simulink model "JointSpaceControl_own_MCP"  (R2013a)
settings: Solver=ode45  StartTime=0.0  StopTime=sim_end  MaxStep=0.008  RelTol=1e-3
PreLoadFcn:
  | Initialization
InitFcn:
  | Initialization
values from neighbouring files (symbols this model uses):
  a_max = [27 27 27 27 27 27]    [Initialization.m]
  dq_0 = qd_actual.signals.values(1,:)    [Initialization.m]
  K_0 = [            omega_1, zeros(1,5);         0,          omega_2, zeros(1,4);         zeros(1,2), omega_3, zeros(1,3);         zeros(1,3), omega_4, zeros(1,2);         zeros(1,4), omega_5, 0;         zeros(1,5), omega_6]    [Initialization.m]
  K_1 = [            omega_7, zeros(1,5);         0,          omega_8, zeros(1,4);         zeros(1,2), omega_9, zeros(1,3);         zeros(1,3), omega_10, zeros(1,2);         zeros(1,4), omega_11, 0;         zeros(1,5), omega_12]    [Initialization.m]
  q_0 = q_actual.signals.values(1,:)    [Initialization.m]
  q_max = 2*pi*ones(1,6)    [Initialization.m]
  q_min = -2*pi*ones(1,6)    [Initialization.m]
  torque_max = [150 150 150 28 28 28]    [Initialization.m]
  v_max = 3.4*ones(1,6)    [Initialization.m]
(part 1 of 4)
settings Model: Creator=kasiunia  LastModifiedBy=kasiunia

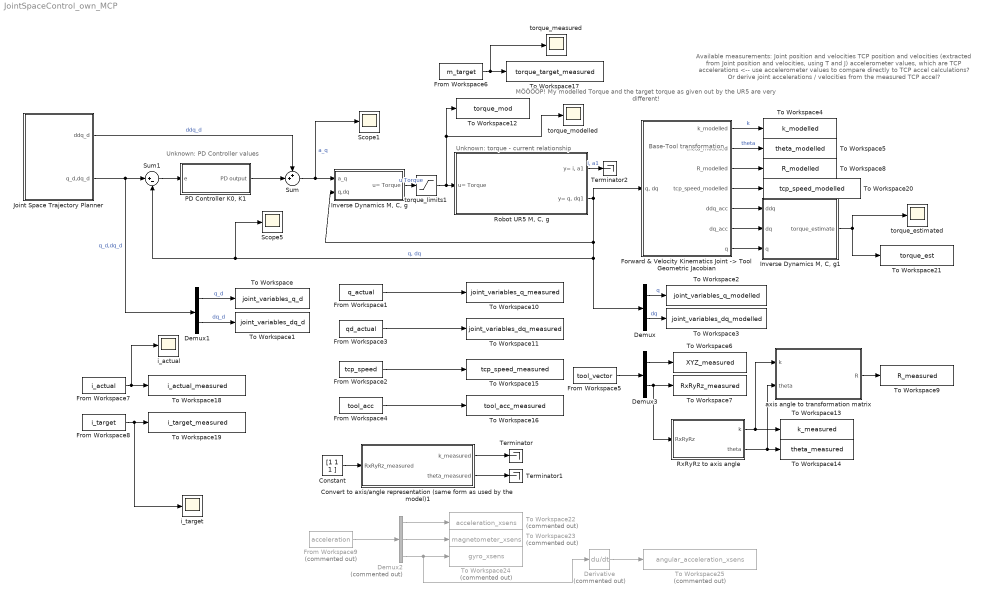
== system JointSpaceControl_own_MCP ==
  note: Base-Tool transformation
  note: Unknown: torque - current relationship
  note: Unknown: PD Controller values
  note: Available measurements:
      | Joint position and velocities
      | TCP position and velocities (extracted from Joint position and velocities,
      | using T and J)
      | accelerometer values, which are TCP accelerations
      | <-- use accelerometer values to compare directly to TCP accel calculations?
      | Or derive joint accelerations / velocities from the measured TCP accel?
  note: MÖÖÖÖP!
      | My modelled Torque and the target torque
      | as given out by the UR5 are very different!
  Constant : Constant  Value=[1 1 1 ]
  Convert to axis/angle representation (same form as used by the model)1 : Subsystem
  Demux : Demux  Outputs=[6 6]
  Demux1 : Demux  Outputs=[6 6]
  Demux2 : Demux  Commented=on  Outputs=[3 3 3]
  Demux3 : Demux  Outputs=[3 3]
  Derivative : Derivative  Commented=on
  "Forward & Velocity Kinematics Joint -> Tool Geometric Jacobian" : Subsystem
  From Workspace1 : FromWorkspace  VariableName=q_actual  SampleTime=0  OutputAfterFinalValue=Holding final value
  From Workspace2 : FromWorkspace  VariableName=tcp_speed  SampleTime=0  OutputAfterFinalValue=Setting to zero
  From Workspace3 : FromWorkspace  VariableName=qd_actual  SampleTime=0  OutputAfterFinalValue=Setting to zero
  From Workspace4 : FromWorkspace  VariableName=tool_acc  SampleTime=0  OutputAfterFinalValue=Setting to zero
  From Workspace5 : FromWorkspace  VariableName=tool_vector  SampleTime=0  OutputAfterFinalValue=Holding final value
  From Workspace6 : FromWorkspace  VariableName=m_target  SampleTime=0  OutputAfterFinalValue=Holding final value
  From Workspace7 : FromWorkspace  VariableName=i_actual  SampleTime=0  OutputAfterFinalValue=Holding final value
  From Workspace8 : FromWorkspace  VariableName=i_target  SampleTime=0  OutputAfterFinalValue=Holding final value
  From Workspace9 : FromWorkspace  Commented=on  VariableName=acceleration  SampleTime=0  OutputAfterFinalValue=Setting to zero
  "Inverse Dynamics M, C, g" : Subsystem
  "Inverse Dynamics M, C, g1" : Subsystem
  Joint Space Trajectory Planner : Subsystem
  "PD Controller K0, K1" : Subsystem
  "Robot UR5 M, C, g" : Subsystem
  RxRyRz to axis angle : MATLAB Function  TreatAsAtomicUnit=on
  Scope1 : Scope
      settings: ShowLegends=on
  Scope5 : Scope
      settings: ShowLegends=on  SaveName=ScopeData4
  Sum : Sum  Inputs=++|
  Sum1 : Sum  Inputs=|+-
  Terminator : Terminator
  Terminator1 : Terminator
  Terminator2 : Terminator
  To Workspace : ToWorkspace  VariableName=joint_variables_q_d  SampleTime=-1  SaveFormat=Timeseries
  To Workspace1 : ToWorkspace  VariableName=joint_variables_dq_d  SampleTime=-1  SaveFormat=Timeseries
  To Workspace10 : ToWorkspace  VariableName=joint_variables_q_measured  SampleTime=-1  SaveFormat=Timeseries
  To Workspace11 : ToWorkspace  VariableName=joint_variables_dq_measured  SampleTime=-1  SaveFormat=Timeseries
  To Workspace12 : ToWorkspace  VariableName=torque_mod  SampleTime=-1  SaveFormat=Timeseries
  To Workspace13 : ToWorkspace  VariableName=k_measured  SampleTime=-1  SaveFormat=Timeseries
  To Workspace14 : ToWorkspace  VariableName=theta_measured  SampleTime=-1  SaveFormat=Timeseries
  To Workspace15 : ToWorkspace  VariableName=tcp_speed_measured  SampleTime=-1  SaveFormat=Timeseries
  To Workspace16 : ToWorkspace  VariableName=tool_acc_measured  SampleTime=-1  SaveFormat=Timeseries
  To Workspace17 : ToWorkspace  VariableName=torque_target_measured  SampleTime=-1  SaveFormat=Timeseries
  To Workspace18 : ToWorkspace  VariableName=i_actual_measured  SampleTime=-1  SaveFormat=Timeseries
  To Workspace19 : ToWorkspace  VariableName=i_target_measured  SampleTime=-1  SaveFormat=Timeseries
  To Workspace2 : ToWorkspace  VariableName=joint_variables_q_modelled  SampleTime=-1  SaveFormat=Timeseries
  To Workspace20 : ToWorkspace  VariableName=tcp_speed_modelled  SampleTime=-1  SaveFormat=Timeseries
  To Workspace21 : ToWorkspace  VariableName=torque_est  SampleTime=-1  SaveFormat=Timeseries
  To Workspace22 : ToWorkspace  Commented=on  VariableName=acceleration_xsens  SampleTime=-1  SaveFormat=Timeseries
  To Workspace23 : ToWorkspace  Commented=on  VariableName=magnetometer_xsens  SampleTime=-1  SaveFormat=Timeseries
  To Workspace24 : ToWorkspace  Commented=on  VariableName=gyro_xsens  SampleTime=-1  SaveFormat=Timeseries
  To Workspace25 : ToWorkspace  Commented=on  VariableName=angular_acceleration_xsens  SampleTime=-1  SaveFormat=Timeseries
  To Workspace3 : ToWorkspace  VariableName=joint_variables_dq_modelled  SampleTime=-1  SaveFormat=Timeseries
  To Workspace4 : ToWorkspace  VariableName=k_modelled  SampleTime=-1  SaveFormat=Timeseries
  To Workspace5 : ToWorkspace  VariableName=theta_modelled  SampleTime=-1  SaveFormat=Timeseries
  To Workspace6 : ToWorkspace  VariableName=XYZ_measured  SampleTime=-1  SaveFormat=Timeseries
  To Workspace7 : ToWorkspace  VariableName=RxRyRz_measured  SampleTime=-1  SaveFormat=Timeseries
  To Workspace8 : ToWorkspace  VariableName=R_modelled  SampleTime=-1  SaveFormat=Timeseries
  To Workspace9 : ToWorkspace  VariableName=R_measured  SampleTime=-1  SaveFormat=Timeseries
  axis angle to transformation matrix : MATLAB Function  TreatAsAtomicUnit=on
  i_actual : Scope
      settings: ShowLegends=on  SaveName=ScopeData12
  i_target : Scope
      settings: SaveName=ScopeData13
  torque_estimated : Scope
      settings: ShowLegends=on  TimeRange=30  SaveName=ScopeData15
  torque_limits1 : Saturate  UpperLimit=torque_max  LowerLimit=-torque_max
  torque_measured : Scope
      settings: ShowLegends=on  TimeRange=50  SaveName=ScopeData16
  torque_modelled : Scope
      settings: ShowLegends=on  TimeRange=27.53110288501713  YMin=-0.9845613223672318  YMax=1.015679985521526  SaveName=ScopeData17
  wires:
  Sum/1 -> "Inverse Dynamics M, C, g"/1(a_q), Scope1/1  "a_q"
  "PD Controller K0, K1"/1(PD output) -> Sum/2
  Joint Space Trajectory Planner/2(q_d,dq_d) -> Sum1/1, Demux1/1  "q_d,dq_d"
  Sum1/1 -> "PD Controller K0, K1"/1(e)
  "Robot UR5 M, C, g"/2("y= q, dq1") -> Demux/1, Scope5/1, Sum1/2, "Inverse Dynamics M, C, g"/2(q,dq), "Forward & Velocity Kinematics Joint -> Tool Geometric Jacobian"/1("q, dq")  "q, dq"
  Joint Space Trajectory Planner/1(ddq_d) -> Sum/1  "ddq_d"
  Demux1/1 -> To Workspace/1  "q_d"
  Demux1/2 -> To Workspace1/1  "dq_d"
  Demux/1 -> To Workspace2/1  "q"
  Demux/2 -> To Workspace3/1  "dq"
  From Workspace5/1 -> Demux3/1
  Demux3/1 -> To Workspace6/1
  Demux3/2 -> RxRyRz to axis angle/1(RxRyRz), To Workspace7/1
  "Forward & Velocity Kinematics Joint -> Tool Geometric Jacobian"/1(k_modelled) -> To Workspace4/1  "k"
  "Forward & Velocity Kinematics Joint -> Tool Geometric Jacobian"/2(theta_modelled) -> To Workspace5/1  "theta"
  RxRyRz to axis angle/1(k) -> axis angle to transformation matrix/1(k), To Workspace13/1
  RxRyRz to axis angle/2(theta) -> axis angle to transformation matrix/2(theta), To Workspace14/1
  Constant/1 -> Convert to axis/angle representation (same form as used by the model)1/1(RxRyRz_measured)
  Convert to axis/angle representation (same form as used by the model)1/1(k_measured) -> Terminator/1
  Convert to axis/angle representation (same form as used by the model)1/2(theta_measured) -> Terminator1/1
  "Forward & Velocity Kinematics Joint -> Tool Geometric Jacobian"/3(R_modelled) -> To Workspace8/1
  axis angle to transformation matrix/1(R) -> To Workspace9/1
  "Robot UR5 M, C, g"/1("y= i, a1") -> Terminator2/1  "i, a1"
  From Workspace2/1 -> To Workspace15/1
  From Workspace4/1 -> To Workspace16/1
  From Workspace6/1 -> torque_measured/1, To Workspace17/1
  From Workspace7/1 -> i_actual/1, To Workspace18/1
  From Workspace8/1 -> i_target/1, To Workspace19/1
  "Forward & Velocity Kinematics Joint -> Tool Geometric Jacobian"/4(tcp_speed_modelled) -> To Workspace20/1
  "Forward & Velocity Kinematics Joint -> Tool Geometric Jacobian"/5(ddq_acc) -> "Inverse Dynamics M, C, g1"/1(ddq)
  "Forward & Velocity Kinematics Joint -> Tool Geometric Jacobian"/6(dq_acc) -> "Inverse Dynamics M, C, g1"/2(dq)
  "Inverse Dynamics M, C, g1"/1(torque_estimate) -> To Workspace21/1, torque_estimated/1
  "Forward & Velocity Kinematics Joint -> Tool Geometric Jacobian"/7(q) -> "Inverse Dynamics M, C, g1"/3(q)
  From Workspace9/1 -> Demux2/1
  Demux2/1 -> To Workspace22/1
  Demux2/2 -> To Workspace23/1
  Demux2/3 -> Derivative/1, To Workspace24/1
  Derivative/1 -> To Workspace25/1
  "Inverse Dynamics M, C, g"/1(u= Torque) -> torque_limits1/1  "u Torque"
  torque_limits1/1 -> torque_modelled/1, To Workspace12/1, "Robot UR5 M, C, g"/1(u= Torque)
  From Workspace1/1 -> To Workspace10/1
  From Workspace3/1 -> To Workspace11/1

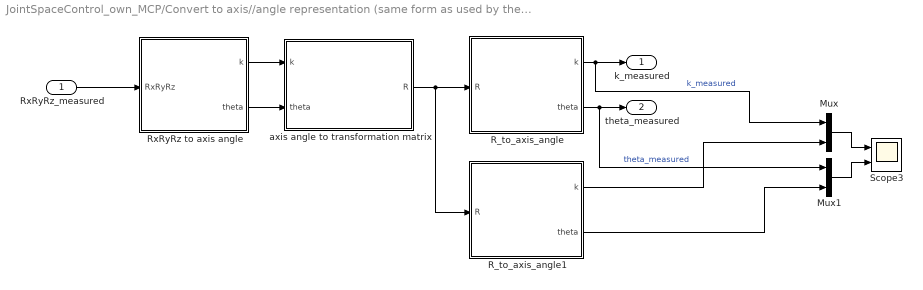
== system JointSpaceControl_own_MCP/Convert to axis//angle representation (same form as used by the model)1 ==
  RxRyRz_measured : Inport
  Mux : Mux  Inputs=[3 3]
  Mux1 : Mux  Inputs=2
  R_to_axis_angle : MATLAB Function  TreatAsAtomicUnit=on
  R_to_axis_angle1 : MATLAB Function  TreatAsAtomicUnit=on
  RxRyRz to axis angle : MATLAB Function  TreatAsAtomicUnit=on
  Scope3 : Scope  NumInputPorts=2
      settings: ShowLegends=on  YMin=-5~-5  YMax=5~5  SaveName=ScopeData6
  axis angle to transformation matrix : MATLAB Function  TreatAsAtomicUnit=on
  k_measured : Outport
  theta_measured : Outport  Port=2
  wires:
  R_to_axis_angle1/2(theta) -> Mux1/2
  R_to_axis_angle1/1(k) -> Mux/2
  Mux1/1 -> Scope3/2
  Mux/1 -> Scope3/1
  RxRyRz_measured/1 -> RxRyRz to axis angle/1(RxRyRz)
  RxRyRz to axis angle/2(theta) -> axis angle to transformation matrix/2(theta)
  RxRyRz to axis angle/1(k) -> axis angle to transformation matrix/1(k)
  R_to_axis_angle/1(k) -> k_measured/1, Mux/1  "k_measured"
  axis angle to transformation matrix/1(R) -> R_to_axis_angle/1(R), R_to_axis_angle1/1(R)
  R_to_axis_angle/2(theta) -> theta_measured/1, Mux1/1  "theta_measured"

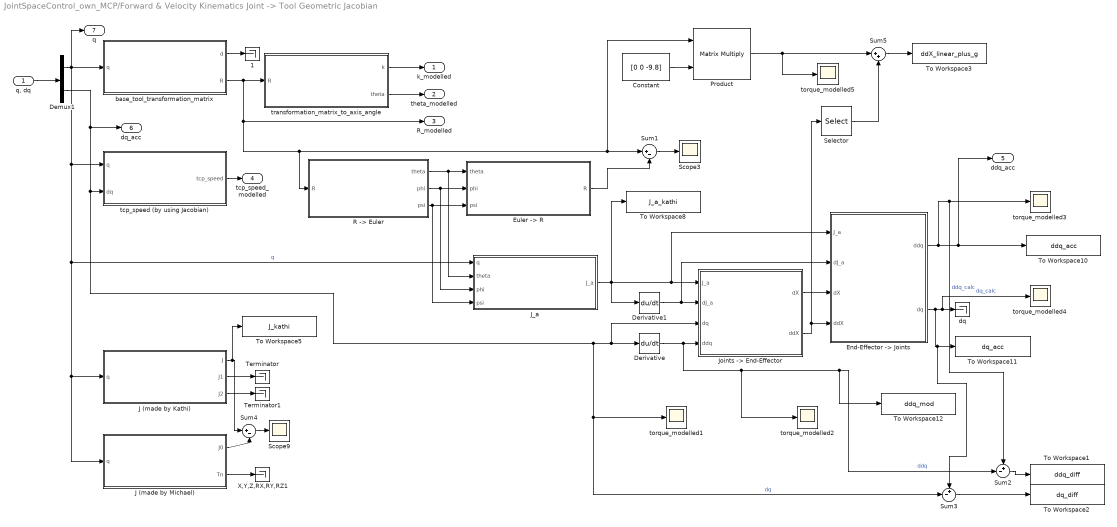
== system JointSpaceControl_own_MCP/Forward & Velocity Kinematics Joint -> Tool Geometric Jacobian ==
  "q, dq" : Inport
  1 : Terminator
  Constant : Constant  Value=[0 0 -9.8]
  Demux1 : Demux  Outputs=[6 6]
  Derivative : Derivative
  Derivative1 : Derivative
  "End-Effector -> Joints" : Subsystem
  "Euler -> R" : MATLAB Function  TreatAsAtomicUnit=on
  J (made by Kathi) : MATLAB Function  TreatAsAtomicUnit=on
  J (made by Michael) : MATLAB Function  TreatAsAtomicUnit=on
  J_a : MATLAB Function  TreatAsAtomicUnit=on
  "Joints -> End-Effector" : Subsystem
  Product : Product  Multiplication=Matrix(*)
  "R -> Euler" : MATLAB Function  TreatAsAtomicUnit=on
  Scope3 : Scope
      settings: ShowLegends=on  SaveName=ScopeData8
  Scope9 : Scope
      settings: ShowLegends=on  SaveName=ScopeData14
  Selector : Selector  InputPortWidth=6  IndexOptions=Index vector (dialog)  Indices=[1 2 3]  OutputSizes=1
  Sum1 : Sum  Inputs=|+-
  Sum2 : Sum  Inputs=+-|
  Sum3 : Sum  Inputs=+-|
  Sum4 : Sum  Inputs=|+-
  Sum5 : Sum  Inputs=|++
  Terminator : Terminator
  Terminator1 : Terminator
  To Workspace1 : ToWorkspace  VariableName=ddq_diff  SampleTime=-1  SaveFormat=Timeseries
  To Workspace10 : ToWorkspace  VariableName=ddq_acc  SampleTime=-1  SaveFormat=Timeseries
  To Workspace11 : ToWorkspace  VariableName=dq_acc  SampleTime=-1  SaveFormat=Timeseries
  To Workspace12 : ToWorkspace  VariableName=ddq_mod  SampleTime=-1  SaveFormat=Timeseries
  To Workspace2 : ToWorkspace  VariableName=dq_diff  SampleTime=-1  SaveFormat=Timeseries
  To Workspace3 : ToWorkspace  VariableName=ddX_linear_plus_g  SampleTime=-1  SaveFormat=Timeseries
  To Workspace5 : ToWorkspace  VariableName=J_kathi  SampleTime=-1  SaveFormat=Timeseries
  To Workspace8 : ToWorkspace  VariableName=J_a_kathi  SampleTime=-1  SaveFormat=Timeseries
  X,Y,Z,RX,RY,RZ1 : Terminator
  base_tool_transformation_matrix : MATLAB Function  TreatAsAtomicUnit=on
  dq : Terminator
  tcp_speed (by using Jacobian) : MATLAB Function  TreatAsAtomicUnit=on
  torque_modelled{1..5} (5 alike) : Scope
      torque_modelled1 settings: ShowLegends=on  SaveName=ScopeData5
      torque_modelled2 settings: ShowLegends=on  SaveName=ScopeData7
      torque_modelled3 settings: ShowLegends=on  SaveName=ScopeData9
      torque_modelled4 settings: ShowLegends=on  SaveName=ScopeData10
      torque_modelled5 settings: ShowLegends=on  SaveName=ScopeData11
  transformation_matrix_to_axis_angle : MATLAB Function  TreatAsAtomicUnit=on
  k_modelled : Outport
  theta_modelled : Outport  Port=2
  R_modelled : Outport  Port=3
  tcp_speed_modelled : Outport  Port=4
  ddq_acc : Outport  Port=5
  dq_acc : Outport  Port=6
  q : Outport  Port=7
  wires:
  "q, dq"/1 -> Demux1/1
  Demux1/1 -> q/1, J (made by Michael)/1(q), J (made by Kathi)/1(q), J_a/1(q), tcp_speed (by using Jacobian)/1(q), base_tool_transformation_matrix/1(q)  "q"
  Demux1/2 -> dq_acc/1, Sum3/2, torque_modelled1/1, "Joints -> End-Effector"/3(dq), Derivative/1, tcp_speed (by using Jacobian)/2(dq)  "dq"
  base_tool_transformation_matrix/2(R) -> transformation_matrix_to_axis_angle/1(R), Product/1, Sum1/1, "R -> Euler"/1(R), R_modelled/1
  transformation_matrix_to_axis_angle/1(k) -> k_modelled/1
  transformation_matrix_to_axis_angle/2(theta) -> theta_modelled/1
  J (made by Kathi)/1(J) -> To Workspace5/1, Sum4/1
  J (made by Michael)/1(J0) -> Sum4/2
  Sum4/1 -> Scope9/1
  J (made by Michael)/2(Tn) -> X,Y,Z,RX,RY,RZ1/1
  tcp_speed (by using Jacobian)/1(tcp_speed) -> tcp_speed_modelled/1
  "R -> Euler"/3(psi) -> J_a/4(psi), "Euler -> R"/3(psi)
  "R -> Euler"/2(phi) -> J_a/3(phi), "Euler -> R"/2(phi)
  "R -> Euler"/1(theta) -> J_a/2(theta), "Euler -> R"/1(theta)
  Sum1/1 -> Scope3/1
  base_tool_transformation_matrix/1(d) -> 1/1
  "Euler -> R"/1(R) -> Sum1/2
  J_a/1(J_a) -> "Joints -> End-Effector"/1(J_a), "End-Effector -> Joints"/1(J_a), To Workspace8/1, Derivative1/1
  Derivative/1 -> torque_modelled2/1, To Workspace12/1, Sum2/2, "Joints -> End-Effector"/4(ddq)  "ddq"
  "Joints -> End-Effector"/2(ddX) -> Selector/1, "End-Effector -> Joints"/4(ddX)
  "Joints -> End-Effector"/1(dX) -> "End-Effector -> Joints"/3(dX)
  Derivative1/1 -> "Joints -> End-Effector"/2(dJ_a), "End-Effector -> Joints"/2(dJ_a)
  "End-Effector -> Joints"/2(dq) -> Sum3/1, To Workspace11/1, torque_modelled4/1, dq/1  "dq_calc"
  J (made by Kathi)/2(J1) -> Terminator/1
  J (made by Kathi)/3(J2) -> Terminator1/1
  "End-Effector -> Joints"/1(ddq) -> torque_modelled3/1, Sum2/1, ddq_acc/1, To Workspace10/1  "ddq_calc"
  Sum2/1 -> To Workspace1/1
  Sum3/1 -> To Workspace2/1
  Constant/1 -> Product/2
  Product/1 -> torque_modelled5/1, Sum5/1
  Selector/1 -> Sum5/2
  Sum5/1 -> To Workspace3/1

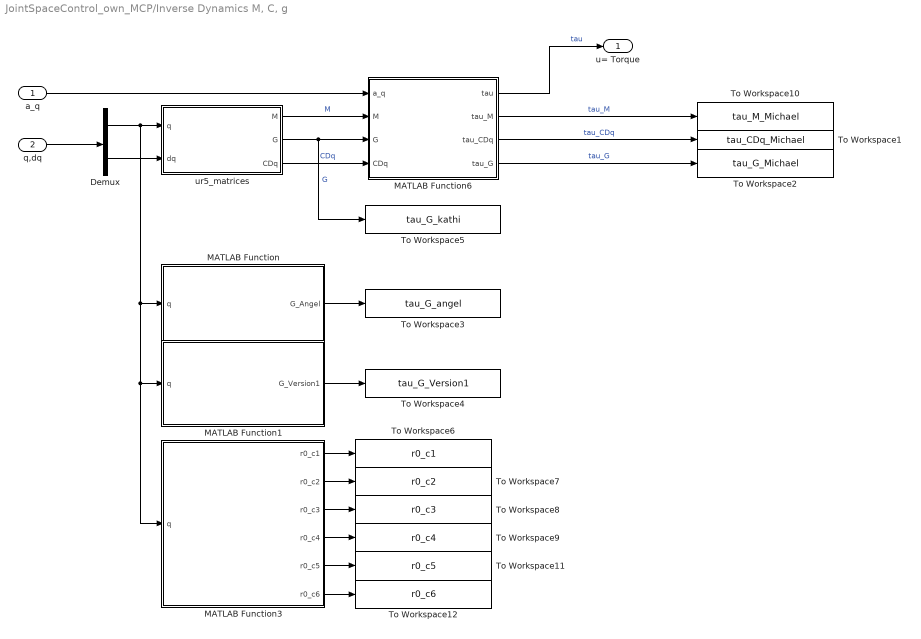
== system JointSpaceControl_own_MCP/Inverse Dynamics M, C, g ==
  a_q : Inport
  q,dq : Inport  Port=2
  Demux : Demux  Outputs=[6 6]
  MATLAB Function : MATLAB Function  TreatAsAtomicUnit=on
  MATLAB Function1 : MATLAB Function  TreatAsAtomicUnit=on
  MATLAB Function3 : MATLAB Function  TreatAsAtomicUnit=on
  MATLAB Function6 : MATLAB Function  TreatAsAtomicUnit=on
  To Workspace1 : ToWorkspace  VariableName=tau_CDq_Michael  SampleTime=-1  SaveFormat=Timeseries
  To Workspace10 : ToWorkspace  VariableName=tau_M_Michael  SampleTime=-1  SaveFormat=Timeseries
  To Workspace11 : ToWorkspace  VariableName=r0_c5  SampleTime=-1  SaveFormat=Timeseries
  To Workspace12 : ToWorkspace  VariableName=r0_c6  SampleTime=-1  SaveFormat=Timeseries
  To Workspace2 : ToWorkspace  VariableName=tau_G_Michael  SampleTime=-1  SaveFormat=Timeseries
  To Workspace3 : ToWorkspace  VariableName=tau_G_angel  SampleTime=-1  SaveFormat=Timeseries
  To Workspace4 : ToWorkspace  VariableName=tau_G_Version1  SampleTime=-1  SaveFormat=Timeseries
  To Workspace5 : ToWorkspace  VariableName=tau_G_kathi  SampleTime=-1  SaveFormat=Timeseries
  To Workspace6 : ToWorkspace  VariableName=r0_c1  SampleTime=-1  SaveFormat=Timeseries
  To Workspace7 : ToWorkspace  VariableName=r0_c2  SampleTime=-1  SaveFormat=Timeseries
  To Workspace8 : ToWorkspace  VariableName=r0_c3  SampleTime=-1  SaveFormat=Timeseries
  To Workspace9 : ToWorkspace  VariableName=r0_c4  SampleTime=-1  SaveFormat=Timeseries
  ur5_matrices : MATLAB Function  TreatAsAtomicUnit=on
  u= Torque : Outport
  wires:
  ur5_matrices/1(M) -> MATLAB Function6/2(M)  "M"
  ur5_matrices/3(CDq) -> MATLAB Function6/4(CDq)  "CDq"
  a_q/1 -> MATLAB Function6/1(a_q)
  Demux/1 -> ur5_matrices/1(q), MATLAB Function3/1(q), MATLAB Function1/1(q), MATLAB Function/1(q)
  Demux/2 -> ur5_matrices/2(dq)
  q,dq/1 -> Demux/1
  MATLAB Function6/1(tau) -> u= Torque/1  "tau"
  MATLAB Function6/2(tau_M) -> To Workspace10/1  "tau_M"
  MATLAB Function6/3(tau_CDq) -> To Workspace1/1  "tau_CDq"
  MATLAB Function6/4(tau_G) -> To Workspace2/1  "tau_G"
  MATLAB Function/1(G_Angel) -> To Workspace3/1
  MATLAB Function1/1(G_Version1) -> To Workspace4/1
  MATLAB Function3/1(r0_c1) -> To Workspace6/1
  MATLAB Function3/2(r0_c2) -> To Workspace7/1
  MATLAB Function3/3(r0_c3) -> To Workspace8/1
  MATLAB Function3/4(r0_c4) -> To Workspace9/1
  MATLAB Function3/5(r0_c5) -> To Workspace11/1
  MATLAB Function3/6(r0_c6) -> To Workspace12/1
  ur5_matrices/2(G) -> To Workspace5/1, MATLAB Function6/3(G)  "G"

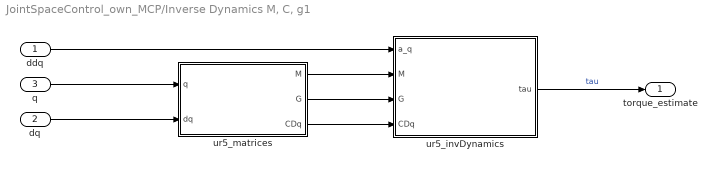
== system JointSpaceControl_own_MCP/Inverse Dynamics M, C, g1 ==
  ddq : Inport
  dq : Inport  Port=2
  q : Inport  Port=3
  ur5_invDynamics : MATLAB Function  TreatAsAtomicUnit=on
  ur5_matrices : MATLAB Function  TreatAsAtomicUnit=on
  torque_estimate : Outport
  wires:
  ur5_invDynamics/1(tau) -> torque_estimate/1  "tau"
  ddq/1 -> ur5_invDynamics/1(a_q)
  ur5_matrices/3(CDq) -> ur5_invDynamics/4(CDq)
  ur5_matrices/2(G) -> ur5_invDynamics/3(G)
  ur5_matrices/1(M) -> ur5_invDynamics/2(M)
  q/1 -> ur5_matrices/1(q)
  dq/1 -> ur5_matrices/2(dq)

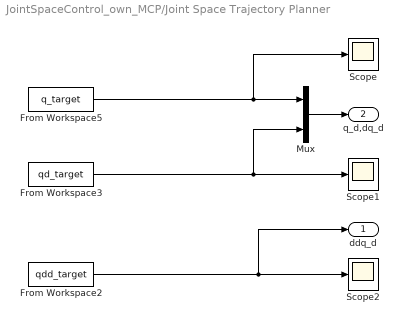
== system JointSpaceControl_own_MCP/Joint Space Trajectory Planner ==
  From Workspace2 : FromWorkspace  VariableName=qdd_target  SampleTime=0  OutputAfterFinalValue=Setting to zero
  From Workspace3 : FromWorkspace  VariableName=qd_target  SampleTime=0  OutputAfterFinalValue=Setting to zero
  From Workspace5 : FromWorkspace  VariableName=q_target  SampleTime=0  OutputAfterFinalValue=Holding final value
  Mux : Mux  Inputs=[6 6]
  Scope : Scope
      settings: ShowLegends=on
  Scope1 : Scope
      settings: ShowLegends=on  SaveName=ScopeData2
  Scope2 : Scope
      settings: ShowLegends=on  SaveName=ScopeData3
  ddq_d : Outport
  q_d,dq_d : Outport  Port=2
  wires:
  Mux/1 -> q_d,dq_d/1
  From Workspace5/1 -> Mux/1, Scope/1
  From Workspace3/1 -> Mux/2, Scope1/1
  From Workspace2/1 -> ddq_d/1, Scope2/1

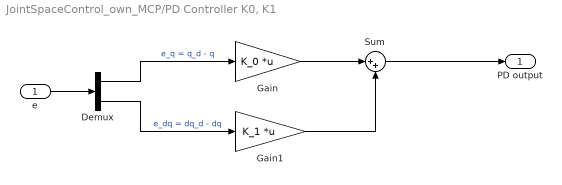
== system JointSpaceControl_own_MCP/PD Controller K0, K1 ==
  e : Inport
  Demux : Demux  Outputs=[6 6]
  Gain : Gain  Gain=K_0  Multiplication=Matrix(K*u) (u vector)
  Gain1 : Gain  Gain=K_1  Multiplication=Matrix(K*u) (u vector)
  Sum : Sum  Inputs=|++
  PD output : Outport
  wires:
  e/1 -> Demux/1
  Sum/1 -> PD output/1
  Demux/1 -> Gain/1  "e_q = q_d - q"
  Demux/2 -> Gain1/1  "e_dq = dq_d - dq"
  Gain1/1 -> Sum/2
  Gain/1 -> Sum/1

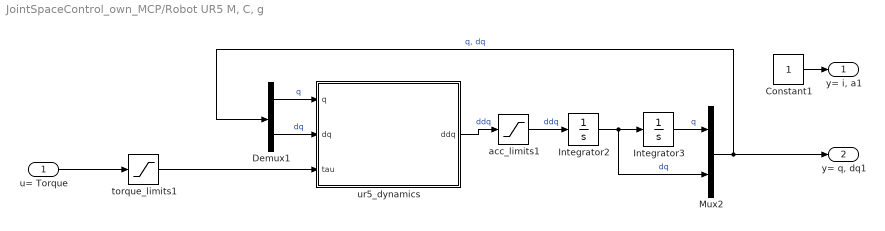
== system JointSpaceControl_own_MCP/Robot UR5 M, C, g ==
  u= Torque : Inport
  Constant1 : Constant
  Demux1 : Demux  Outputs=[6 6]
  Integrator2 : Integrator  InitialCondition=[dq_0]  LimitOutput=on  UpperSaturationLimit=v_max  LowerSaturationLimit=-v_max  ContinuousStateAttributes='velocity'
  Integrator3 : Integrator  InitialCondition=[q_0]  LimitOutput=on  UpperSaturationLimit=q_max  LowerSaturationLimit=q_min  ContinuousStateAttributes='position'
  Mux2 : Mux  Inputs=[6 6]
  acc_limits1 : Saturate  UpperLimit=a_max  LowerLimit=-a_max
  torque_limits1 : Saturate  UpperLimit=torque_max  LowerLimit=-torque_max
  ur5_dynamics : MATLAB Function  TreatAsAtomicUnit=on
  "y= i, a1" : Outport
  "y= q, dq1" : Outport  Port=2
  wires:
  ur5_dynamics/1(ddq) -> acc_limits1/1  "ddq"
  Integrator2/1 -> Integrator3/1, Mux2/2  "dq"
  Integrator3/1 -> Mux2/1  "q"
  Mux2/1 -> "y= q, dq1"/1, Demux1/1  "q, dq"
  Constant1/1 -> "y= i, a1"/1
  Demux1/1 -> ur5_dynamics/1(q)  "q"
  Demux1/2 -> ur5_dynamics/2(dq)  "dq"
  acc_limits1/1 -> Integrator2/1  "ddq"
  torque_limits1/1 -> ur5_dynamics/3(tau)
  u= Torque/1 -> torque_limits1/1

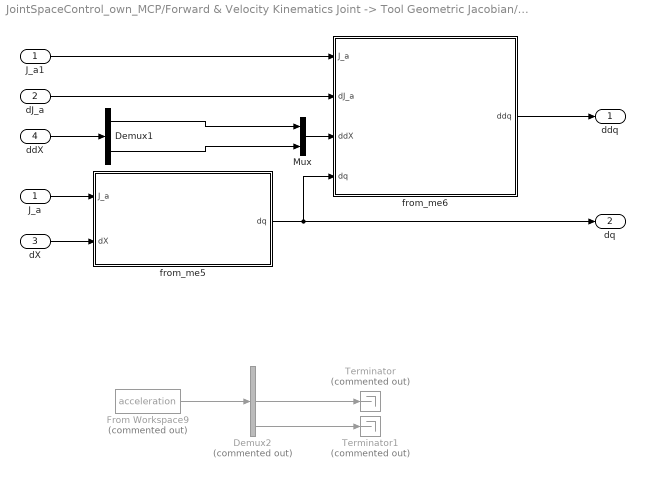
== system JointSpaceControl_own_MCP/Forward & Velocity Kinematics Joint -> Tool Geometric Jacobian/End-Effector -> Joints ==
  J_a : Inport
  dJ_a : Inport  Port=2
  dX : Inport  Port=3
  ddX : Inport  Port=4
  Demux1 : Demux  Outputs=[3 3]
  Demux2 : Demux  Commented=on  Outputs=[3 3 3]
  From Workspace9 : FromWorkspace  Commented=on  VariableName=acceleration  SampleTime=0  OutputAfterFinalValue=Setting to zero
  J_a1 : InportShadow
  Mux : Mux  Inputs=[3 3]
  Terminator : Terminator  Commented=on
  Terminator1 : Terminator  Commented=on
  from_me5 : MATLAB Function  TreatAsAtomicUnit=on
  from_me6 : MATLAB Function  TreatAsAtomicUnit=on
  ddq : Outport
  dq : Outport  Port=2
  wires:
  from_me6/1(ddq) -> ddq/1
  J_a/1 -> from_me5/1(J_a)
  J_a1/1 -> from_me6/1(J_a)
  dJ_a/1 -> from_me6/2(dJ_a)
  dX/1 -> from_me5/2(dX)
  from_me5/1(dq) -> dq/1, from_me6/4(dq)
  From Workspace9/1 -> Demux2/1
  Demux2/2 -> Terminator/1
  Demux2/3 -> Terminator1/1
  Mux/1 -> from_me6/3(ddX)
  Demux1/2 -> Mux/2
  ddX/1 -> Demux1/1
  Demux1/1 -> Mux/1

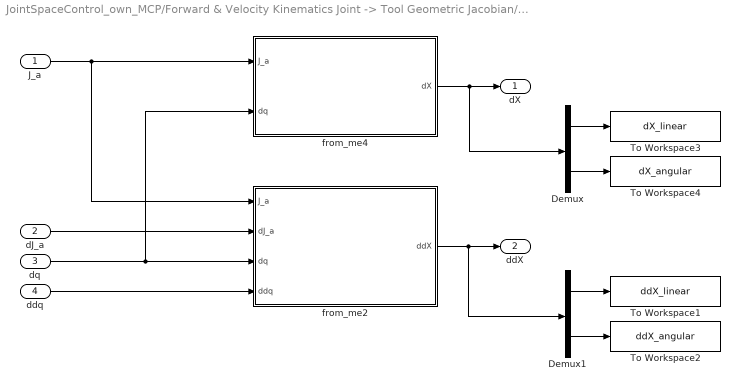
== system JointSpaceControl_own_MCP/Forward & Velocity Kinematics Joint -> Tool Geometric Jacobian/Joints -> End-Effector ==
  J_a : Inport
  dJ_a : Inport  Port=2
  dq : Inport  Port=3
  ddq : Inport  Port=4
  Demux : Demux  Outputs=[3 3]
  Demux1 : Demux  Outputs=[3 3]
  To Workspace1 : ToWorkspace  VariableName=ddX_linear  SampleTime=-1  SaveFormat=Timeseries
  To Workspace2 : ToWorkspace  VariableName=ddX_angular  SampleTime=-1  SaveFormat=Timeseries
  To Workspace3 : ToWorkspace  VariableName=dX_linear  SampleTime=-1  SaveFormat=Timeseries
  To Workspace4 : ToWorkspace  VariableName=dX_angular  SampleTime=-1  SaveFormat=Timeseries
  from_me2 : MATLAB Function  TreatAsAtomicUnit=on
  from_me4 : MATLAB Function  TreatAsAtomicUnit=on
  dX : Outport
  ddX : Outport  Port=2
  wires:
  from_me4/1(dX) -> Demux/1, dX/1
  from_me2/1(ddX) -> Demux1/1, ddX/1
  J_a/1 -> from_me2/1(J_a), from_me4/1(J_a)
  dJ_a/1 -> from_me2/2(dJ_a)
  dq/1 -> from_me4/2(dq), from_me2/3(dq)
  ddq/1 -> from_me2/4(ddq)
  Demux/1 -> To Workspace3/1
  Demux/2 -> To Workspace4/1
  Demux1/1 -> To Workspace1/1
  Demux1/2 -> To Workspace2/1

== matlab function JointSpaceControl_own_MCP/Inverse Dynamics M, C, g/ur5_matrices ==
  data: q input; M output; dq input; G output; CDq output
function [ M, G, CDq ] = ur5_Matrices( q, dq)
%#codegen
%Returns the acceleration of the manipulator based on its dynamics
[ M, G, CDq ] = ur5_matrices( q, dq );

== matlab function JointSpaceControl_own_MCP/Inverse Dynamics M, C, g/MATLAB Function3 ==
  data: q input; r0_c1 output; r0_c2 output; r0_c3 output; r0_c4 output; r0_c5 output; r0_c6 output
function [r0_c1, r0_c2, r0_c3, r0_c4, r0_c5, r0_c6]  = UR5_r0ci(q)
%#codegen
%Returns the dynamics of the UR5 manipulator

theta_1 = q(1);
theta_2 = q(2);
theta_3 = q(3);
theta_4 = q(4);
theta_5 = q(5);
theta_6 = q(6);

r1_c1 = [0, -0.02561, 0.00193];
r2_c2 = [0.2125, 0, 0.11336];
r3_c3 = [0.11993, 0, 0.0265];
r4_c4 = [0, -0.0018, 0.01634];
r5_c5 = [0, 0.0018,0.01634];
r6_c6 = [0, 0, -0.001159];

 
R1 = [cos(theta_1), 0,  sin(theta_1); ...
      sin(theta_1), 0, -cos(theta_1); ...
      0,            1,             0];
R2 = [cos(theta_1)*cos(theta_2), -cos(theta_1)*sin(theta_2),  sin(theta_1); ...
      cos(theta_2)*sin(theta_1), -sin(theta_1)*sin(theta_2), -cos(theta_1); ...
      sin(theta_2),               cos(theta_2),             0];
R3 = [cos(theta_1)*cos(theta_2)*cos(theta_3) - cos(theta_1)*sin(theta_2)*sin(theta_3), - cos(theta_1)*cos(theta_2)*sin(theta_3) - cos(theta_1)*cos(theta_3)*sin(theta_2),  sin(theta_1); ...
      cos(theta_2)*cos(theta_3)*sin(theta_1) - sin(theta_1)*sin(theta_2)*sin(theta_3), - cos(theta_2)*sin(theta_1)*sin(theta_3) - cos(theta_3)*sin(theta_1)*sin(theta_2), -cos(theta_1);
      cos(theta_2)*sin(theta_3) + cos(theta_3)*sin(theta_2),                             cos(theta_2)*cos(theta_3) - sin(theta_2)*sin(theta_3),             0];
R4 = [- cos(theta_4)*(cos(theta_1)*sin(theta_2)*sin(theta_3) - cos(theta_1)*cos(theta_2)*cos(theta_3)) - sin(theta_4)*(cos(theta_1)*cos(theta_2)*sin(theta_3) + cos(theta_1)*cos(theta_3)*sin(theta_2)),  sin(theta_1), cos(theta_4)*(cos(theta_1)*cos(theta_2)*sin(theta_3) + cos(theta_1)*cos(theta_3)*sin(theta_2)) - sin(theta_4)*(cos(theta_1)*sin(theta_2)*sin(theta_3) - cos(theta_1)*cos(theta_2)*cos(theta_3)); ...
      - cos(theta_4)*(sin(theta_1)*sin(theta_2)*sin(theta_3) - cos(theta_2)*cos(theta_3)*sin(theta_1)) - sin(theta_4)*(cos(theta_2)*sin(theta_1)*sin(theta_3) + cos(theta_3)*sin(theta_1)*sin(theta_2)), -cos(theta_1), cos(theta_4)*(cos(theta_2)*sin(theta_1)*sin(theta_3) + cos(theta_3)*sin(theta_1)*sin(theta_2)) - sin(theta_4)*(sin(theta_1)*sin(theta_2)*sin(theta_3) - cos(theta_2)*cos(theta_3)*sin(theta_1)); ...
      cos(theta_4)*(cos(theta_2)*sin(theta_3) + cos(theta_3)*sin(theta_2)) + sin(theta_4)*(cos(theta_2)*cos(theta_3) - sin(theta_2)*sin(theta_3)),             0,                                                     sin(theta_4)*(cos(theta_2)*sin(theta_3) + cos(theta_3)*sin(theta_2)) - cos(theta_4)*(cos(theta_2)*cos(theta_3) - sin(theta_2)*sin(theta_3))]; 
R5 = [   sin(theta_1)*sin(theta_5) - cos(theta_5)*(cos(theta_4)*(cos(theta_1)*sin(theta_2)*sin(theta_3) - cos(theta_1)*cos(theta_2)*cos(theta_3)) + sin(theta_4)*(cos(theta_1)*cos(theta_2)*sin(theta_3) + cos(theta_1)*cos(theta_3)*sin(theta_2))), sin(theta_4)*(cos(theta_1)*sin(theta_2)*sin(theta_3) - cos(theta_1)*cos(theta_2)*cos(theta_3)) - cos(theta_4)*(cos(theta_1)*cos(theta_2)*sin(theta_3) + cos(theta_1)*cos(theta_3)*sin(theta_2)), cos(theta_5)*sin(theta_1) + sin(theta_5)*(cos(theta_4)*(cos(theta_1)*sin(theta_2)*sin(theta_3) - cos(theta_1)*cos(theta_2)*cos(theta_3)) + sin(theta_4)*(cos(theta_1)*cos(theta_2)*sin(theta_3) + cos(theta_1)*cos(theta_3)*sin(theta_2))); ...
      - cos(theta_1)*sin(theta_5) - cos(theta_5)*(cos(theta_4)*(sin(theta_1)*sin(theta_2)*sin(theta_3) - cos(theta_2)*cos(theta_3)*sin(theta_1)) + sin(theta_4)*(cos(theta_2)*sin(theta_1)*sin(theta_3) + cos(theta_3)*sin(theta_1)*sin(theta_2))), sin(theta_4)*(sin(theta_1)*sin(theta_2)*sin(theta_3) - cos(theta_2)*cos(theta_3)*sin(theta_1)) - cos(theta_4)*(cos(theta_2)*sin(theta_1)*sin(theta_3) + cos(theta_3)*sin(theta_1)*sin(theta_2)), sin(theta_5)*(cos(theta_4)*(sin(theta_1)*sin(theta_2)*sin(theta_3) - cos(theta_2)*cos(theta_3)*sin(theta_1)) + sin(theta_4)*(cos(theta_2)*sin(theta_1)*sin(theta_3) + cos(theta_3)*sin(theta_1)*sin(theta_2))) - cos(theta_1)*cos(theta_5); ...
      cos(theta_5)*(cos(theta_4)*(cos(theta_2)*sin(theta_3) + cos(theta_3)*sin(theta_2)) + sin(theta_4)*(cos(theta_2)*cos(theta_3) - sin(theta_2)*sin(theta_3))),                                                     cos(theta_4)*(cos(theta_2)*cos(theta_3) - sin(theta_2)*sin(theta_3)) - sin(theta_4)*(cos(theta_2)*sin(theta_3) + cos(theta_3)*sin(theta_2)),                                                                                -sin(theta_5)*(cos(theta_4)*(cos(theta_2)*sin(theta_3) + cos(theta_3)*sin(theta_2)) + sin(theta_4)*(cos(theta_2)*cos(theta_3) - sin(theta_2)*sin(theta_3)))]; 
R6 = [   cos(theta_6)*(sin(theta_1)*sin(theta_5) - cos(theta_5)*(cos(theta_4)*(cos(theta_1)*sin(theta_2)*sin(theta_3) - cos(theta_1)*cos(theta_2)*cos(theta_3)) + sin(theta_4)*(cos(theta_1)*cos(theta_2)*sin(theta_3) + cos(theta_1)*cos(theta_3)*sin(theta_2)))) - sin(theta_6)*(cos(theta_4)*(cos(theta_1)*cos(theta_2)*sin(theta_3) + cos(theta_1)*cos(theta_3)*sin(theta_2)) - sin(theta_4)*(cos(theta_1)*sin(theta_2)*sin(theta_3) - cos(theta_1)*cos(theta_2)*cos(theta_3))), - sin(theta_6)*(sin(theta_1)*sin(theta_5) - cos(theta_5)*(cos(theta_4)*(cos(theta_1)*sin(theta_2)*sin(theta_3) - cos(theta_1)*cos(theta_2)*cos(theta_3)) + sin(theta_4)*(cos(theta_1)*cos(theta_2)*sin(theta_3) + cos(theta_1)*cos(theta_3)*sin(theta_2)))) - cos(theta_6)*(cos(theta_4)*(cos(theta_1)*cos(theta_2)*sin(theta_3) + cos(theta_1)*cos(theta_3)*sin(theta_2)) - sin(theta_4)*(cos(theta_1)*sin(theta_2)*sin(theta_3) - cos(theta_1)*cos(theta_2)*cos(theta_3))), cos(theta_5)*sin(theta_1) + sin(theta_5)*(cos(theta_4)*(cos(theta_1)*sin(theta_2)*sin(theta_3) - cos(theta_1)*cos(theta_2)*cos(theta_3)) + sin(theta_4)*(cos(theta_1)*cos(theta_2)*sin(theta_3) + cos(theta_1)*cos(theta_3)*sin(theta_2))); ...
      - cos(theta_6)*(cos(theta_1)*sin(theta_5) + cos(theta_5)*(cos(theta_4)*(sin(theta_1)*sin(theta_2)*sin(theta_3) - cos(theta_2)*cos(theta_3)*sin(theta_1)) + sin(theta_4)*(cos(theta_2)*sin(theta_1)*sin(theta_3) + cos(theta_3)*sin(theta_1)*sin(theta_2)))) - sin(theta_6)*(cos(theta_4)*(cos(theta_2)*sin(theta_1)*sin(theta_3) + cos(theta_3)*sin(theta_1)*sin(theta_2)) - sin(theta_4)*(sin(theta_1)*sin(theta_2)*sin(theta_3) - cos(theta_2)*cos(theta_3)*sin(theta_1))),   sin(theta_6)*(cos(theta_1)*sin(theta_5) + cos(theta_5)*(cos(theta_4)*(sin(theta_1)*sin(theta_2)*sin(theta_3) - cos(theta_2)*cos(theta_3)*sin(theta_1)) + sin(theta_4)*(cos(theta_2)*sin(theta_1)*sin(theta_3) + cos(theta_3)*sin(theta_1)*sin(theta_2)))) - cos(theta_6)*(cos(theta_4)*(cos(theta_2)*sin(theta_1)*sin(theta_3) + cos(theta_3)*sin(theta_1)*sin(theta_2)) - sin(theta_4)*(sin(theta_1)*sin(theta_2)*sin(theta_3) - cos(theta_2)*cos(theta_3)*sin(theta_1))), sin(theta_5)*(cos(theta_4)*(sin(theta_1)*sin(theta_2)*sin(theta_3) - cos(theta_2)*cos(theta_3)*sin(theta_1)) + sin(theta_4)*(cos(theta_2)*sin(theta_1)*sin(theta_3) + cos(theta_3)*sin(theta_1)*sin(theta_2))) - cos(theta_1)*cos(theta_5); ...
      sin(theta_6)*(cos(theta_4)*(cos(theta_2)*cos(theta_3) - sin(theta_2)*sin(theta_3)) - sin(theta_4)*(cos(theta_2)*sin(theta_3) + cos(theta_3)*sin(theta_2))) + cos(theta_5)*cos(theta_6)*(cos(theta_4)*(cos(theta_2)*sin(theta_3) + cos(theta_3)*sin(theta_2)) + sin(theta_4)*(cos(theta_2)*cos(theta_3) - sin(theta_2)*sin(theta_3))),                                                                                                                                         cos(theta_6)*(cos(theta_4)*(cos(theta_2)*cos(theta_3) - sin(theta_2)*sin(theta_3)) - sin(theta_4)*(cos(theta_2)*sin(theta_3) + cos(theta_3)*sin(theta_2))) - cos(theta_5)*sin(theta_6)*(cos(theta_4)*(cos(theta_2)*sin(theta_3) + cos(theta_3)*sin(theta_2)) + sin(theta_4)*(cos(theta_2)*cos(theta_3) - sin(theta_2)*sin(theta_3))),                                                                                -sin(theta_5)*(cos(theta_4)*(cos(theta_2)*sin(theta_3) + cos(theta_3)*sin(theta_2)) + sin(theta_4)*(cos(theta_2)*cos(theta_3) - sin(theta_2)*sin(theta_3)))];
 
d1 = [ 0; 0; 223/2500];
d2 = [  -(17*cos(theta_1)*cos(theta_2))/40; ...
      -(17*cos(theta_2)*sin(theta_1))/40; ...
      223/2500 - (17*sin(theta_2))/40];
d3 = [ (39243*cos(theta_1)*sin(theta_2)*sin(theta_3))/100000 - (17*cos(theta_1)*cos(theta_2))/40 - (39243*cos(theta_1)*cos(theta_2)*cos(theta_3))/100000; ...
    (39243*sin(theta_1)*sin(theta_2)*sin(theta_3))/100000 - (17*cos(theta_2)*sin(theta_1))/40 - (39243*cos(theta_2)*cos(theta_3)*sin(theta_1))/100000; ...
    223/2500 - (39243*cos(theta_2)*sin(theta_3))/100000 - (39243*cos(theta_3)*sin(theta_2))/100000 - (17*sin(theta_2))/40];
d4 = [ (109*sin(theta_1))/1000 - (17*cos(theta_1)*cos(theta_2))/40 + (39243*cos(theta_1)*sin(theta_2)*sin(theta_3))/100000 - (39243*cos(theta_1)*cos(theta_2)*cos(theta_3))/100000; ...
    (39243*sin(theta_1)*sin(theta_2)*sin(theta_3))/100000 - (17*cos(theta_2)*sin(theta_1))/40 - (109*cos(theta_1))/1000 - (39243*cos(theta_2)*cos(theta_3)*sin(theta_1))/100000; ...
    223/2500 - (39243*cos(theta_2)*sin(theta_3))/100000 - (39243*cos(theta_3)*sin(theta_2))/100000 - (17*sin(theta_2))/40];
d5 = [ (109*sin(theta_1))/1000 - (17*cos(theta_1)*cos(theta_2))/40 + (93*cos(theta_4)*(cos(theta_1)*cos(theta_2)*sin(theta_3) + cos(theta_1)*cos(theta_3)*sin(theta_2)))/1000 - (93*sin(theta_4)*(cos(theta_1)*sin(theta_2)*sin(theta_3) - cos(theta_1)*cos(theta_2)*cos(theta_3)))/1000 + (39243*cos(theta_1)*sin(theta_2)*sin(theta_3))/100000 - (39243*cos(theta_1)*cos(theta_2)*cos(theta_3))/100000; ...
    (93*cos(theta_4)*(cos(theta_2)*sin(theta_1)*sin(theta_3) + cos(theta_3)*sin(theta_1)*sin(theta_2)))/1000 - (17*cos(theta_2)*sin(theta_1))/40 - (109*cos(theta_1))/1000 - (93*sin(theta_4)*(sin(theta_1)*sin(theta_2)*sin(theta_3) - cos(theta_2)*cos(theta_3)*sin(theta_1)))/1000 + (39243*sin(theta_1)*sin(theta_2)*sin(theta_3))/100000 - (39243*cos(theta_2)*cos(theta_3)*sin(theta_1))/100000; ...
    (93*sin(theta_4)*(cos(theta_2)*sin(theta_3) + cos(theta_3)*sin(theta_2)))/1000 - (39243*cos(theta_2)*sin(theta_3))/100000 - (39243*cos(theta_3)*sin(theta_2))/100000 - (93*cos(theta_4)*(cos(theta_2)*cos(theta_3) - sin(theta_2)*sin(theta_3)))/1000 - (17*sin(theta_2))/40 + 223/2500];
d6 = [ (109*sin(theta_1))/1000 - (17*cos(theta_1)*cos(theta_2))/40 + (41*cos(theta_5)*sin(theta_1))/500 + (93*cos(theta_4)*(cos(theta_1)*cos(theta_2)*sin(theta_3) + cos(theta_1)*cos(theta_3)*sin(theta_2)))/1000 - (93*sin(theta_4)*(cos(theta_1)*sin(theta_2)*sin(theta_3) - cos(theta_1)*cos(theta_2)*cos(theta_3)))/1000 + (41*sin(theta_5)*(cos(theta_4)*(cos(theta_1)*sin(theta_2)*sin(theta_3) - cos(theta_1)*cos(theta_2)*cos(theta_3)) + sin(theta_4)*(cos(theta_1)*cos(theta_2)*sin(theta_3) + cos(theta_1)*cos(theta_3)*sin(theta_2))))/500 + (39243*cos(theta_1)*sin(theta_2)*sin(theta_3))/100000 - (39243*cos(theta_1)*cos(theta_2)*cos(theta_3))/100000; ...
    (93*cos(theta_4)*(cos(theta_2)*sin(theta_1)*sin(theta_3) + cos(theta_3)*sin(theta_1)*sin(theta_2)))/1000 - (41*cos(theta_1)*cos(theta_5))/500 - (17*cos(theta_2)*sin(theta_1))/40 - (109*cos(theta_1))/1000 - (93*sin(theta_4)*(sin(theta_1)*sin(theta_2)*sin(theta_3) - cos(theta_2)*cos(theta_3)*sin(theta_1)))/1000 + (41*sin(theta_5)*(cos(theta_4)*(sin(theta_1)*sin(theta_2)*sin(theta_3) - cos(theta_2)*cos(theta_3)*sin(theta_1)) + sin(theta_4)*(cos(theta_2)*sin(theta_1)*sin(theta_3) + cos(theta_3)*sin(theta_1)*sin(theta_2))))/500 + (39243*sin(theta_1)*sin(theta_2)*sin(theta_3))/100000 - (39243*cos(theta_2)*cos(theta_3)*sin(theta_1))/100000; ...
    (93*sin(theta_4)*(cos(theta_2)*sin(theta_3) + cos(theta_3)*sin(theta_2)))/1000 - (39243*cos(theta_2)*sin(theta_3))/100000 - (39243*cos(theta_3)*sin(theta_2))/100000 - (41*sin(theta_5)*(cos(theta_4)*(cos(theta_2)*sin(theta_3) + cos(theta_3)*sin(theta_2)) + sin(theta_4)*(cos(theta_2)*cos(theta_3) - sin(theta_2)*sin(theta_3))))/500 - (93*cos(theta_4)*(cos(theta_2)*cos(theta_3) - sin(theta_2)*sin(theta_3)))/1000 - (17*sin(theta_2))/40 + 223/2500];


r0_c1 = d1 + R1*r1_c1';
r0_c2 = d2 + R2*r2_c2';
r0_c3 = d3 + R3*r3_c3';
r0_c4 = d4 + R4*r4_c4';
r0_c5 = d5 + R5*r5_c5';
r0_c6 = d6 + R6*r6_c6';


end

== matlab function JointSpaceControl_own_MCP/Inverse Dynamics M, C, g1/ur5_matrices ==
  data: q input; M output; dq input; G output; CDq output
function [ M, G, CDq ] = ur5_Matrices( q, dq)
%#codegen
%Returns the acceleration of the manipulator based on its dynamics
[ M, G, CDq ] = ur5_matrices( q, dq );

== matlab function JointSpaceControl_own_MCP/Forward & Velocity Kinematics Joint -> Tool Geometric Jacobian/R -> Euler ==
  data: theta output; phi output; R input; psi output
function [theta, phi, psi]  = R_to_euler_angle(R)
%R_TO_EULER_ANGLE Transform rotation matrix to euler-angle format, where
%the rotation happens around ZYZ, with R_ZYZ = R_Z,phi*R_Y,theta*R_Z,psi
r_11 = R(1,1);
r_12 = R(1,2);
r_13 = R(1,3);
r_21 = R(2,1);
r_22 = R(2,2);
r_23 = R(2,3);
r_31 = R(3,1);
r_32 = R(3,2);
r_33 = R(3,3);

if (r_13 ~= 0) || (r_23 ~= 0)
    theta = atan2(sqrt(r_13^2+r_23^2),r_33);
    phi = atan2(r_23, r_13);
    psi = atan2(r_32, -r_31);
elseif (r_13 == 0) && (r_23 == 0)
    if (r_33 == 1)
        theta = 0;
        phi = 0;
        psi = atan2(r_11, r_21) - phi;
    elseif (r_33 == -1)
        theta = pi;
        phi = 0;
        psi = -(atan2(-r_11, -r_12) - phi);
    else
        error('r_33 must be +1 or -1')
    end
else
    error('Make sure that the values are almost equal zero')
end
end

== matlab function JointSpaceControl_own_MCP/Forward & Velocity Kinematics Joint -> Tool Geometric Jacobian/transformation_matrix_to_axis_angle ==
  data: k output; R input; theta output
function [k, theta]  = R_to_axis_angle(R)
%BaseToolTransformationMatrix - Transformationmatrix from Base to Tool
%  Calculates the Base-Tool Transformation matrix based on the current
%  joint positions.
 theta = acos((R(1,1)+R(2,2)+R(3,3)-1)/2);
 k = 1/(2*sin(theta))*[R(3,2)-R(2,3); R(1,3)-R(3,1); R(2,1)-R(1,2)];
end

== matlab function JointSpaceControl_own_MCP/RxRyRz to axis angle ==
  data: RxRyRz input; k output; theta output
function [k, theta]  = RxRyRz_to_k_theta(RxRyRz)
% RXRYRZ_TO_K_THETA Transform the RxRyRz representation to the axis/angle
% representation
 theta = norm(RxRyRz);
 k = RxRyRz/theta;
end

== matlab function JointSpaceControl_own_MCP/axis angle to transformation matrix ==
  data: k input; theta input; R output
function R   = axis_angle_to_R(k, theta)
% AXIS_ANGLE_TO_R Transform the axis/angle representation to a rotation
% matrix representation.
kx = k(1);
ky = k(2);
kz = k(3);

v = 1-cos(theta);
s = sin(theta);
c = cos (theta);

r11 = kx^2*v + c;
r12 = kx*ky*v - kz*s;
r13 = kx*kz*v+ky*s;
r21 = kx*ky*v+kz*s;
r22 = ky^2*v + c;
r23 = ky*kz*v-kx*s;
r31 = kx*kz*v-ky*s;
r32 = ky*kz*v + kx*s;
r33 = kz^2*v+c;

R = [r11, r12, r13; r21, r22, r23; r31, r32, r33];

end

== matlab function JointSpaceControl_own_MCP/Forward & Velocity Kinematics Joint -> Tool Geometric Jacobian/tcp_speed (by using Jacobian) ==
  data: tcp_speed output; q input; dq input
function tcp_speed     = tcp_speed(q, dq)
% JACOBIAN - Jacobian from Base to Tool.
%  Calculates the Base-Tool Transformation matrix based on the current
%  joint positions and returns the rotation matrix and the displacement
%  vector.

theta_1 = q(1);
theta_2 = q(2);
theta_3 = q(3);
theta_4 = q(4);
theta_5 = q(5);
theta_6 = q(6);

J = [(109*cos(theta_1))/1000 + (41*cos(theta_1)*cos(theta_5))/500 + ...
        (17*cos(theta_2)*sin(theta_1))/40 - ...
        (93*cos(theta_4)*(cos(theta_2)*sin(theta_1)*sin(theta_3) + ...
        cos(theta_3)*sin(theta_1)*sin(theta_2)))/1000 + ...
        (93*sin(theta_4)*(sin(theta_1)*sin(theta_2)*sin(theta_3) - ...
        cos(theta_2)*cos(theta_3)*sin(theta_1)))/1000 - ...
        (41*sin(theta_5)*(cos(theta_4)*(sin(theta_1)*sin(theta_2)*sin(theta_3) - ...
        cos(theta_2)*cos(theta_3)*sin(theta_1)) + ...
        sin(theta_4)*(cos(theta_2)*sin(theta_1)*sin(theta_3) + ...
        cos(theta_3)*sin(theta_1)*sin(theta_2))))/500 - ...
        (39243*sin(theta_1)*sin(theta_2)*sin(theta_3))/100000 + ...
        (39243*cos(theta_2)*cos(theta_3)*sin(theta_1))/100000, ...
        ...
        (17*cos(theta_1)*sin(theta_2))/40 - ...
        (93*cos(theta_4)*(cos(theta_1)*sin(theta_2)*sin(theta_3) - ...
        cos(theta_1)*cos(theta_2)*cos(theta_3)))/1000 - ...
        (93*sin(theta_4)*(cos(theta_1)*cos(theta_2)*sin(theta_3) + ...
        cos(theta_1)*cos(theta_3)*sin(theta_2)))/1000 + ...
        (41*sin(theta_5)*(cos(theta_4)*(cos(theta_1)*cos(theta_2)*sin(theta_3) + ...
        cos(theta_1)*cos(theta_3)*sin(theta_2)) - ...
        sin(theta_4)*(cos(theta_1)*sin(theta_2)*sin(theta_3) - ...
        cos(theta_1)*cos(theta_2)*cos(theta_3))))/500 + ...
        (39243*cos(theta_1)*cos(theta_2)*sin(theta_3))/100000 + ...
        (39243*cos(theta_1)*cos(theta_3)*sin(theta_2))/100000, ...
        ...
        (41*sin(theta_5)*(cos(theta_4)*(cos(theta_1)*cos(theta_2)*sin(theta_3) + ...
        cos(theta_1)*cos(theta_3)*sin(theta_2)) - ...
        sin(theta_4)*(cos(theta_1)*sin(theta_2)*sin(theta_3) - ...
        cos(theta_1)*cos(theta_2)*cos(theta_3))))/500 - ...
        (93*sin(theta_4)*(cos(theta_1)*cos(theta_2)*sin(theta_3) + ...
        cos(theta_1)*cos(theta_3)*sin(theta_2)))/1000 - ...
        (93*cos(theta_4)*(cos(theta_1)*sin(theta_2)*sin(theta_3) - ...
        cos(theta_1)*cos(theta_2)*cos(theta_3)))/1000 + ...
        (39243*cos(theta_1)*cos(theta_2)*sin(theta_3))/100000 + ...
        (39243*cos(theta_1)*cos(theta_3)*sin(theta_2))/100000, ...
        ...
        (41*sin(theta_5)*(cos(theta_4)*(cos(theta_1)*cos(theta_2)*sin(theta_3) + ...
        cos(theta_1)*cos(theta_3)*sin(theta_2)) - ...
        sin(theta_4)*(cos(theta_1)*sin(theta_2)*sin(theta_3) - ...
        cos(theta_1)*cos(theta_2)*cos(theta_3))))/500 - ...
        (93*sin(theta_4)*(cos(theta_1)*cos(theta_2)*sin(theta_3) + ...
        cos(theta_1)*cos(theta_3)*sin(theta_2)))/1000 - ...
        (93*cos(theta_4)*(cos(theta_1)*sin(theta_2)*sin(theta_3) - ...
        cos(theta_1)*cos(theta_2)*cos(theta_3)))/1000, ...
        ...
        (41*cos(theta_5)*(cos(theta_4)*(cos(theta_1)*sin(theta_2)*sin(theta_3) - ...
        cos(theta_1)*cos(theta_2)*cos(theta_3)) + ...
        sin(theta_4)*(cos(theta_1)*cos(theta_2)*sin(theta_3) + ...
        cos(theta_1)*cos(theta_3)*sin(theta_2))))/500 - ...
        (41*sin(theta_1)*sin(theta_5))/500,... 
        ...
        0; ...
   (109*sin(theta_1))/1000 - (17*cos(theta_1)*cos(theta_2))/40 + ...
        (41*cos(theta_5)*sin(theta_1))/500 + ...
        (93*cos(theta_4)*(cos(theta_1)*cos(theta_2)*sin(theta_3) + ...
        cos(theta_1)*cos(theta_3)*sin(theta_2)))/1000 - ...
        (93*sin(theta_4)*(cos(theta_1)*sin(theta_2)*sin(theta_3) - ... 
        cos(theta_1)*cos(theta_2)*cos(theta_3)))/1000 + ...
        (41*sin(theta_5)*(cos(theta_4)*(cos(theta_1)*sin(theta_2)*sin(theta_3) - ...
        cos(theta_1)*cos(theta_2)*cos(theta_3)) + ...
        sin(theta_4)*(cos(theta_1)*cos(theta_2)*sin(theta_3) + ...
        cos(theta_1)*cos(theta_3)*sin(theta_2))))/500 + ...
        (39243*cos(theta_1)*sin(theta_2)*sin(theta_3))/100000 - ...
        (39243*cos(theta_1)*cos(theta_2)*cos(theta_3))/100000, ...
        ...
        (17*sin(theta_1)*sin(theta_2))/40 - ...
        (93*cos(theta_4)*(sin(theta_1)*sin(theta_2)*sin(theta_3) - ...
        cos(theta_2)*cos(theta_3)*sin(theta_1)))/1000 - ...
        (93*sin(theta_4)*(cos(theta_2)*sin(theta_1)*sin(theta_3) + ...
        cos(theta_3)*sin(theta_1)*sin(theta_2)))/1000 + ...
        (41*sin(theta_5)*(cos(theta_4)*(cos(theta_2)*sin(theta_1)*sin(theta_3) + ...
        cos(theta_3)*sin(theta_1)*sin(theta_2)) - ...
        sin(theta_4)*(sin(theta_1)*sin(theta_2)*sin(theta_3) - ...
        cos(theta_2)*cos(theta_3)*sin(theta_1))))/500 + ...
        (39243*cos(theta_2)*sin(theta_1)*sin(theta_3))/100000 + ...
        (39243*cos(theta_3)*sin(theta_1)*sin(theta_2))/100000, ...
        ...
        (41*sin(theta_5)*(cos(theta_4)*(cos(theta_2)*sin(theta_1)*sin(theta_3) + ...
        cos(theta_3)*sin(theta_1)*sin(theta_2)) - ...
        sin(theta_4)*(sin(theta_1)*sin(theta_2)*sin(theta_3) - ...
        cos(theta_2)*cos(theta_3)*sin(theta_1))))/500 - ...
        (93*sin(theta_4)*(cos(theta_2)*sin(theta_1)*sin(theta_3) + ...
        cos(theta_3)*sin(theta_1)*sin(theta_2)))/1000 - ...
        (93*cos(theta_4)*(sin(theta_1)*sin(theta_2)*sin(theta_3) - ...
        cos(theta_2)*cos(theta_3)*sin(theta_1)))/1000 + ...
        (39243*cos(theta_2)*sin(theta_1)*sin(theta_3))/100000 + ...
        (39243*cos(theta_3)*sin(theta_1)*sin(theta_2))/100000, ...
        ...
        (41*sin(theta_5)*(cos(theta_4)*(cos(theta_2)*sin(theta_1)*sin(theta_3) + ...
        cos(theta_3)*sin(theta_1)*sin(theta_2)) - ...
        sin(theta_4)*(sin(theta_1)*sin(theta_2)*sin(theta_3) - ...
        cos(theta_2)*cos(theta_3)*sin(theta_1))))/500 - ...
        (93*sin(theta_4)*(cos(theta_2)*sin(theta_1)*sin(theta_3) + ...
        cos(theta_3)*sin(theta_1)*sin(theta_2)))/1000 - ...
        (93*cos(theta_4)*(sin(theta_1)*sin(theta_2)*sin(theta_3) - ...
        cos(theta_2)*cos(theta_3)*sin(theta_1)))/1000, ...
        ...
        (41*cos(theta_1)*sin(theta_5))/500 + ...
        (41*cos(theta_5)*(cos(theta_4)*(sin(theta_1)*sin(theta_2)*sin(theta_3) - ...
        cos(theta_2)*cos(theta_3)*sin(theta_1)) + ...
        sin(theta_4)*(cos(theta_2)*sin(theta_1)*sin(theta_3) + ...
        cos(theta_3)*sin(theta_1)*sin(theta_2))))/500, ...
        ...
        0; ...
    0, ...
        ...
        (39243*sin(theta_2)*sin(theta_3))/100000 - ...
        (39243*cos(theta_2)*cos(theta_3))/100000 - ...
        (17*cos(theta_2))/40 - ...
        (41*sin(theta_5)*(cos(theta_4)*(cos(theta_2)*cos(theta_3) - ...
        sin(theta_2)*sin(theta_3)) - sin(theta_4)*(cos(theta_2)*sin(theta_3) + ...
        cos(theta_3)*sin(theta_2))))/500 + ...
        (93*cos(theta_4)*(cos(theta_2)*sin(theta_3) + ...
        cos(theta_3)*sin(theta_2)))/1000 + ...
        (93*sin(theta_4)*(cos(theta_2)*cos(theta_3) - sin(theta_2)*sin(theta_3)))/1000,...
        ...
        (39243*sin(theta_2)*sin(theta_3))/100000 - ...
        (39243*cos(theta_2)*cos(theta_3))/100000 - ...
        (41*sin(theta_5)*(cos(theta_4)*(cos(theta_2)*cos(theta_3) - ...
        sin(theta_2)*sin(theta_3)) - sin(theta_4)*(cos(theta_2)*sin(theta_3) + ...
        cos(theta_3)*sin(theta_2))))/500 + (93*cos(theta_4)*(cos(theta_2)*sin(theta_3) + ...
        cos(theta_3)*sin(theta_2)))/1000 + (93*sin(theta_4)*(cos(theta_2)*cos(theta_3) - ...
        sin(theta_2)*sin(theta_3)))/1000, ...
        ...
        (93*cos(theta_4)*(cos(theta_2)*sin(theta_3) + cos(theta_3)*sin(theta_2)))/1000 - ...
        (41*sin(theta_5)*(cos(theta_4)*(cos(theta_2)*cos(theta_3) - ...
        sin(theta_2)*sin(theta_3)) - sin(theta_4)*(cos(theta_2)*sin(theta_3) + ...
        cos(theta_3)*sin(theta_2))))/500 + (93*sin(theta_4)*(cos(theta_2)*cos(theta_3) - ...
        sin(theta_2)*sin(theta_3)))/1000,  ...
        ...
        -(41*cos(theta_5)*(cos(theta_4)*(cos(theta_2)*sin(theta_3) + ...
        cos(theta_3)*sin(theta_2)) + sin(theta_4)*(cos(theta_2)*cos(theta_3) - ...
        sin(theta_2)*sin(theta_3))))/500,  ...
        ...
        0; ...
    0, ...
        ...
        sin(theta_1), ...
        ...
        sin(theta_1), ...
        ...
        sin(theta_1), ...
        ...
        cos(theta_4)*(cos(theta_1)*cos(theta_2)*sin(theta_3) + ...
        cos(theta_1)*cos(theta_3)*sin(theta_2)) - ...
        sin(theta_4)*(cos(theta_1)*sin(theta_2)*sin(theta_3) - ...
        cos(theta_1)*cos(theta_2)*cos(theta_3)), ...
        ...
        cos(theta_5)*sin(theta_1) + ...
        sin(theta_5)*(cos(theta_4)*(cos(theta_1)*sin(theta_2)*sin(theta_3) - ...
        cos(theta_1)*cos(theta_2)*cos(theta_3)) + ...
        sin(theta_4)*(cos(theta_1)*cos(theta_2)*sin(theta_3) + ...
        cos(theta_1)*cos(theta_3)*sin(theta_2)));...
    0, ...
        ...
        -cos(theta_1), ...
        ...
        -cos(theta_1), ...
        ...
        -cos(theta_1), ...
        ...
        cos(theta_4)*(cos(theta_2)*sin(theta_1)*sin(theta_3) + ...
        cos(theta_3)*sin(theta_1)*sin(theta_2)) - ...
        sin(theta_4)*(sin(theta_1)*sin(theta_2)*sin(theta_3) - ...
        cos(theta_2)*cos(theta_3)*sin(theta_1)), ...
        ...
        sin(theta_5)*(cos(theta_4)*(sin(theta_1)*sin(theta_2)*sin(theta_3) - ...
        cos(theta_2)*cos(theta_3)*sin(theta_1)) + ...
        sin(theta_4)*(cos(theta_2)*sin(theta_1)*sin(theta_3) + ...
        cos(theta_3)*sin(theta_1)*sin(theta_2))) - cos(theta_1)*cos(theta_5);
    1, ...
        ...
        0, ...
        ...
        0, ...
        ...
        0, ...
        ...
        sin(theta_4)*(cos(theta_2)*sin(theta_3) + cos(theta_3)*sin(theta_2)) - ...
        cos(theta_4)*(cos(theta_2)*cos(theta_3) - sin(theta_2)*sin(theta_3)),...
        ...
        -sin(theta_5)*(cos(theta_4)*(cos(theta_2)*sin(theta_3) + ...
        cos(theta_3)*sin(theta_2)) + sin(theta_4)*(cos(theta_2)*cos(theta_3) - ...
        sin(theta_2)*sin(theta_3)));];
    
    tcp_speed = J*dq;

end
